simulink model "Nieliniowy"  (R2018a)
settings: Solver=ode45  StartTime=0.0  StopTime=200  RelTol=1e-3  AbsTol=1e-6  EnableMultiTasking=on
values from neighbouring files (symbols this model uses):
  A1 = 1    [PrzeplywWody.m]    (also in testttt.m)
  A2 = 1    [PrzeplywWody.m]    (also in testttt.m)
  Aw1 = 0.1    [PrzeplywWody.m]    (also in testttt.m)
  Aw2 = 0.2    [PrzeplywWody.m]    (also in testttt.m)
  fwe1 = 1    [PrzeplywWody.m]    (also in testttt.m = 3)
  g = 9.81    [PrzeplywWody.m]    (also in testttt.m)
  h10 = 0    [PrzeplywWody.m]    (also in testttt.m = 3)
  h20 = 0    [PrzeplywWody.m]    (also in testttt.m = 1)
settings Model: Creator=LAB320-1552  LastModifiedBy=john
settings SolverCC: AutoScaleAbsTol=off
settings DataIOCC: LimitDataPoints=on  SaveFormat=Array
settings OptimizationCC: LifeSpan=inf
settings DebuggingCC: UnderspecifiedInitializationDetection=Classic  MergeDetectMultiDrivingBlocksExec=none  StateNameClashWarn=warning  StrictBusMsg=ErrorOnBusTreatedAsVector  SFUnexpectedBacktrackingDiag=warning  SFNoUnconditionalDefaultTransitionDiag=warning  SFExecutionAtInitializationDiag=none
settings HardwareCC: ProdBitPerPointer=32  ProdBitPerSizeT=32  ProdBitPerPtrDiffT=32  ProdLargestAtomicFloat=None  ProdIntDivRoundTo=Undefined  ProdEndianess=Unspecified  ProdWordSize=32  ProdHWDeviceType=32-bit Generic
settings ModelReferenceCC: PropagateSignalLabelsOutOfModel=off
settings CodeAppCC: StateflowObjectComments=on
settings GRTTargetCC: TargetLangStandard=C89/C90 (ANSI)  GeneratePreprocessorConditionals=Disable all
settings ConfigComp: CovMetricSettings=dw  CovHtmlReporting=on  CovSaveCumulativeToWorkspaceVar=on  CovSaveSingleToWorkspaceVar=on  CovExternalEMLEnable=off

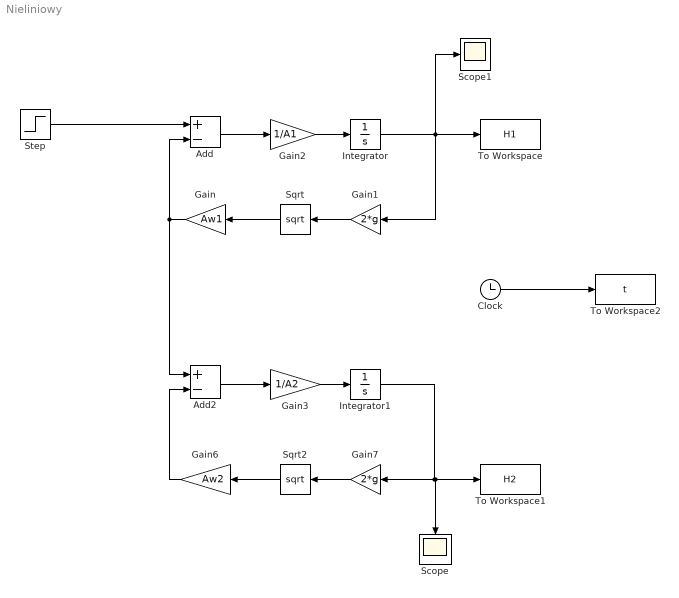
== system Nieliniowy ==
  Add : Sum  Inputs=+-
  Add2 : Sum  Inputs=+-
  Clock : Clock
  Gain : Gain  Gain=Aw1
  Gain1 : Gain  Gain=2*g
  Gain2 : Gain  Gain=1/A1
  Gain3 : Gain  Gain=1/A2
  Gain6 : Gain  Gain=Aw2
  Gain7 : Gain  Gain=2*g
  Integrator : Integrator  InitialCondition=h10
  Integrator1 : Integrator  InitialCondition=h20
  Scope : Scope
  Scope1 : Scope
  Sqrt : Sqrt  SaturateOnIntegerOverflow=on
  Sqrt2 : Sqrt  SaturateOnIntegerOverflow=on
  Step : Step  Time=3  Before=fwe1  After=fwe1+1  SampleTime=0
  To Workspace : ToWorkspace  VariableName=H1  SampleTime=-1
  To Workspace1 : ToWorkspace  VariableName=H2  SampleTime=-1
  To Workspace2 : ToWorkspace  VariableName=t  SampleTime=-1
  wires:
  Step/1 -> Add/1
  Add/1 -> Gain2/1
  Gain2/1 -> Integrator/1
  Gain1/1 -> Sqrt/1
  Sqrt/1 -> Gain/1
  Gain/1 -> Add/2, Add2/1
  Integrator/1 -> Scope1/1, Gain1/1, To Workspace/1
  Add2/1 -> Gain3/1
  Gain3/1 -> Integrator1/1
  Integrator1/1 -> Scope/1, To Workspace1/1, Gain7/1
  Gain7/1 -> Sqrt2/1
  Sqrt2/1 -> Gain6/1
  Clock/1 -> To Workspace2/1
  Gain6/1 -> Add2/2
